simulink library "platooning_custom_blocks"  (R2018b)
settings: Solver=VariableStepAuto  StartTime=0.0  StopTime=10.0  RelTol=1e-3
undefined symbols (not defined in the file): AccPdl_pdlbpt, AccPdl_spdbpt, AccPdl_trqMap, adj_motEffMap, BETModel, BrkPdl_brkTrq, BrkPdl_pdlbpt, Cd_Map, Cd_Map_T2, CT_accPdl_pdlbpt, CT_accPdl_spdbpt, CT_accPdl_trqMap, CT_brkPdl_brkTrq, CT_brkPdl_pdlbpt, CTModel, d_11, d_22, DiscIntNeverNeededParam, init_veh_spd_mps, max_Cd_frac, min_Cd_frac, motSpdVec, motTrqVec, msk_init_pos_m, msk_mot_cont_trq, msk_mot_num, msk_mot_spd_bpt, N_OptResults, sim_t_step, simDrv, SPHETModel, t_step
libraries: simulink x19, $bdroot x16, dspstat3 x2, custom_func x1
(part 4 of 5)

== system platooning_custom_blocks/Series Parallel Hybrid Electric Truck/Series Parallel Hybrid Electric Post-Processing/Distance to Empty Calculator ==
  note: Assuming 10% of the fuel in the tank
      | is not available for consumption.
  blndEC_Wh_m : Inport
  <fuelUsed_L> : Inport  Port=2
  battSOC_frac : Inport  Port=3
  Battery Energy Max : Constant  Value=msk_batt_Ns * msk_batt_Np * msk_batt_Nmod * msk_cell_Vnom * msk_cell_Q_Ah
  Constant : Constant  Value=msk_fuel_init_liters
  Constant1 : Constant  Value=0.2
  Divide : Product  Inputs=*/
  Fuel LHV energy per volume : Constant  Value=msk_fuel_rho_kgpl * msk_fuel_lhv_kwhpkg
  Percent of Fuel in Tank : Gain  Gain=0.9
  Product2 : Product
  Product3 : Product
  Subtract : Sum  Inputs=-+
  Subtract1 : Sum  Inputs=+-
  Subtract2 : Sum  Inputs=++|
  kWh2Wh : Gain  Gain=1000
  m2km : Gain  Gain=0.001
  estDTE_km : Outport
  wires:
  Divide/1 -> m2km/1
  Subtract2/1 -> Divide/1
  kWh2Wh/1 -> Subtract2/2
  Product3/1 -> Subtract2/1
  Subtract1/1 -> Product3/1
  Battery Energy Max/1 -> Product3/2
  Product2/1 -> kWh2Wh/1
  Fuel LHV energy per volume/1 -> Product2/1
  battSOC_frac/1 -> Subtract1/1
  Constant1/1 -> Subtract1/2
  Percent of Fuel in Tank/1 -> Subtract/2
  blndEC_Wh_m/1 -> Divide/2
  <fuelUsed_L>/1 -> Subtract/1
  Subtract/1 -> Product2/2
  Constant/1 -> Percent of Fuel in Tank/1
  m2km/1 -> estDTE_km/1  "estDTE_km"

== system platooning_custom_blocks/Series Parallel Hybrid Electric Truck/Series Parallel Hybrid Electric Post-Processing/Fuel Consumption Calculator ==
  <fuelUsed_L> : Inport
  <DistTrvld_m> : Inport  Port=2
  Constant : Constant  Value=100
  Constant1 : Constant  Value=eps
  Divide1 : Product  Inputs=*/
  Divide2 : Product  Inputs=*/
  Switch : Switch  Criteria=u2 > Threshold
  m2km : Gain  Gain=1/1000
  FC_Lp100km : Outport
  wires:
  Divide2/1 -> FC_Lp100km/1  "FC_Lp100km"
  <DistTrvld_m>/1 -> m2km/1
  Switch/1 -> Divide1/1
  Divide1/1 -> Divide2/2
  m2km/1 -> Switch/1, Switch/2
  <fuelUsed_L>/1 -> Divide1/2
  Constant1/1 -> Switch/3
  Constant/1 -> Divide2/1

== system platooning_custom_blocks/Series Parallel Hybrid Electric Truck/Series Parallel Hybrid Electric Powertrain Power Loss Model/A123 ESS Model ==
  Inp_Current : Inport
  Add : Sum  Inputs=++++
  Bus Creator : BusCreator  Inputs=7
  OCV_Battery : Subsystem
  R0 Resistance : Subsystem
  R1_C1 Circuit : Subsystem
  R2_C2 Circuit : Subsystem
  Info : Outport
  Load_Voltage : Outport  Port=2
  SOC : Outport  Port=3
  Current : Outport  Port=4
  wires:
  [SOC] -> Bus Creator/3
  [U_PA] -> Bus Creator/7
  Inp_Current/1 -> OCV_Battery/1(Current)
  [current] -> Bus Creator/2
  Add/1 -> Load_Voltage/1, [V_L]  "V_L"
  [Em] -> Bus Creator/4
  R0 Resistance/1(V_R0) -> [V_R0], Add/3  "V_R0"
  R2_C2 Circuit/1(U_PA) -> Add/1, [U_PA]  "U_PA"
  OCV_Battery/2(Current_pt) -> Current/1, [current], R2_C2 Circuit/2(Current), R1_C1 Circuit/2(Current), R0 Resistance/2(Current)  "Current"
  OCV_Battery/1(SOC_calc) -> SOC/1, [SOC], R2_C2 Circuit/1(SOC), R1_C1 Circuit/1(SOC), R0 Resistance/1(SOC)  "SOC"
  R1_C1 Circuit/1(U_PC) -> Add/2, [U_PC]  "U_PC"
  [U_PC] -> Bus Creator/6
  OCV_Battery/3(BattVolt_calc) -> [Em], Add/4  "Em"
  [V_R0] -> Bus Creator/5
  Bus Creator/1 -> Info/1  "Info"
  [V_L] -> Bus Creator/1

== system platooning_custom_blocks/Series Parallel Hybrid Electric Truck/Series Parallel Hybrid Electric Powertrain Power Loss Model/Battery EPO Logic ==
  note: Discharge Current is negative
  Batt_SOC_frac : Inport
  LoadCurrent_A : Inport  Port=2
  10-second average : dspstat3/Moving Average  Method=Sliding window  ForgettingFactorPort=off  SpecifyWindowLength=on  WindowLength=1000  ForgettingFactor=0.9  SimulateUsing=Code generation
  10sec Discharge Limit Table A123 : Lookup_n-D  BreakpointsForDimension1=msk_cellTempbpt  BreakpointsForDimension2=msk_soc_bpt  Table=msk_dchglim10s  ExtrapMethod=Clip  UseLastTableValue=on  InternalRulePriority=Speed  RndMeth=Simplest  InputSameDT=on
  Battery EPO Constraint Logic : Stateflow chart  TreatAsAtomicUnit=on
  CellTemp degC : Constant  Value=35
  Gain1 : Gain  Gain=-1
  Batt_EPO : Outport
  wires:
  Batt_SOC_frac/1 -> 10sec Discharge Limit Table A123/2
  LoadCurrent_A/1 -> 10-second average/1
  Battery EPO Constraint Logic/1(epo_flag) -> Batt_EPO/1  "Batt_EPO"
  10-second average/1 -> Battery EPO Constraint Logic/2(LoadCurr)  "LoadCurrent_10sAvg_A"
  CellTemp degC/1 -> 10sec Discharge Limit Table A123/1
  Gain1/1 -> Battery EPO Constraint Logic/1(DchgCurrLim)
  10sec Discharge Limit Table A123/1 -> Gain1/1

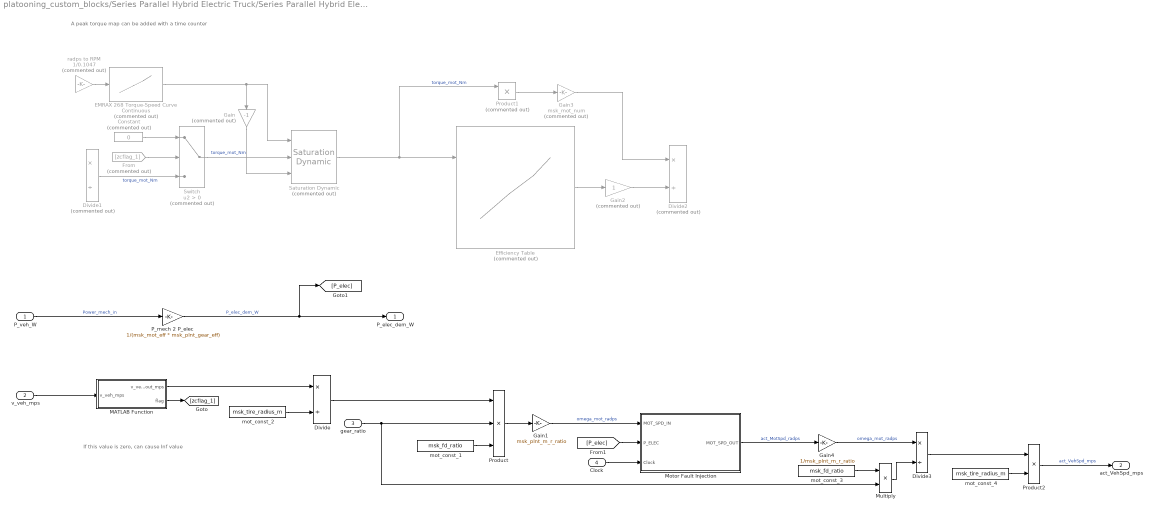
== system platooning_custom_blocks/Series Parallel Hybrid Electric Truck/Series Parallel Hybrid Electric Powertrain Power Loss Model/Electric Drivetrain ==
  note: A peak torque map can be added with a time counter
  note: If this value is zero, can cause Inf value
  P_veh_W : Inport
  v_veh_mps : Inport  Port=2
  gear_ratio : Inport  Port=3
  Clock : Inport  Port=4
  Constant : Constant  Commented=on  Value=0
  Divide : Product  Inputs=*/
  Divide1 : Product  Commented=on  Inputs=*/
  Divide2 : Product  Commented=on  Inputs=*/
  Divide3 : Product  Inputs=*/
  EMRAX 268 Torque-Speed Curve Continuous : Lookup_n-D  Commented=on  NumberOfTableDimensions=1  BreakpointsForDimension1=msk_mot_spd_bpt  Table=msk_mot_cont_trq  InternalRulePriority=Speed  RndMeth=Simplest  InputSameDT=on
  Efficiency Table : Lookup_n-D  Commented=on  BreakpointsForDimension1=motTrqVec  BreakpointsForDimension2=motSpdVec  Table=adj_motEffMap  ExtrapMethod=Clip  UseLastTableValue=on  InternalRulePriority=Speed  RndMeth=Simplest  InputSameDT=on
  From : From  Commented=on  GotoTag=zcflag_1
  Gain : Gain  Commented=on  Gain=-1
  Gain1 : Gain  Gain=msk_plnt_m_r_ratio
  Gain2 : Gain  Commented=on
  Gain3 : Gain  Commented=on  Gain=msk_mot_num
  Gain4 : Gain  Gain=1/msk_plnt_m_r_ratio
  MATLAB Function : MATLAB Function  TreatAsAtomicUnit=on
  Motor Fault Injection : Subsystem  mask{FaultDec=off, P_derate=30000, t_fault=6000, contMotTrqMax=180}
      mask prompts: FaultDec "Select to enable motor deration fault."; P_derate "Enter the motor deration power [Watts]:"; t_fault "Time for fault insertion [seconds]:"; contMotTrqMax "Maximum Continuous Motor Torque [Nm]:"
      mask DialogControl DescGroupVar Prompt: Motor Fault Injection
      mask DialogControl DescTextVar Prompt: Use the parameter controls to induce a deration fault in the motor subsystem.
  Multiply : Product
  P_mech 2 P_elec : Gain  Gain=1/(msk_mot_eff * msk_plnt_gear_eff)
  Product : Product  Inputs=3
  Product1 : Product  Commented=on
  Product2 : Product
  Saturation Dynamic : simulink/Discontinuities/Saturation Dynamic  Commented=on  OutMin=[]  OutMax=[]  OutDataTypeStr=Inherit: Same as second input  OutDataType=fixdt(1, 16)  OutScaling=2^-10  DoSatur=off
  Switch : Switch  Commented=on  Criteria=u2 > Threshold
  mot_const_1 : Constant  Value=msk_fd_ratio
  mot_const_2 : Constant  Value=msk_tire_radius_m
  mot_const_3 : Constant  Value=msk_fd_ratio
  mot_const_4 : Constant  Value=msk_tire_radius_m
  radps to RPM : Gain  Commented=on  Gain=1/0.1047
  P_elec_dem_W : Outport
  act_VehSpd_mps : Outport  Port=2
  wires:
  Saturation Dynamic/1 -> Product1/1, Efficiency Table/1  "torque_mot_Nm"
  From/1 -> Switch/2
  MATLAB Function/1(v_veh_out_mps) -> Divide/1
  radps to RPM/1 -> EMRAX 268 Torque-Speed Curve Continuous/1
  Constant/1 -> Switch/1
  Gain/1 -> Saturation Dynamic/3
  gear_ratio/1 -> Multiply/2, Product/2
  EMRAX 268 Torque-Speed Curve Continuous/1 -> Gain/1, Saturation Dynamic/1
  P_veh_W/1 -> P_mech 2 P_elec/1  "Power_mech_in"
  v_veh_mps/1 -> MATLAB Function/1(v_veh_mps)
  Efficiency Table/1 -> Gain2/1
  Switch/1 -> Saturation Dynamic/2  "torque_mot_Nm"
  mot_const_2/1 -> Divide/2
  MATLAB Function/2(flag) -> [zcflag_1]
  Product1/1 -> Gain3/1
  P_mech 2 P_elec/1 -> [P_elec], P_elec_dem_W/1  "P_elec_dem_W"
  Gain2/1 -> Divide2/2
  Gain3/1 -> Divide2/1
  Divide1/1 -> Switch/3  "torque_mot_Nm"
  Motor Fault Injection/1(MOT_SPD_OUT) -> Gain4/1  "act_MotSpd_radps"
  Gain1/1 -> Motor Fault Injection/1(MOT_SPD_IN)  "omega_mot_radps"
  [P_elec] -> Motor Fault Injection/2(P_ELEC)
  Clock/1 -> Motor Fault Injection/3(Clock)
  mot_const_3/1 -> Multiply/1
  Divide3/1 -> Product2/1
  mot_const_4/1 -> Product2/2
  Product2/1 -> act_VehSpd_mps/1  "act_VehSpd_mps"
  Divide/1 -> Product/1
  mot_const_1/1 -> Product/3
  Product/1 -> Gain1/1
  Gain4/1 -> Divide3/1  "omega_mot_radps"
  Multiply/1 -> Divide3/2

== system platooning_custom_blocks/Series Parallel Hybrid Electric Truck/Series Parallel Hybrid Electric Powertrain Power Loss Model/Engine Torque Saturation ==
  eng_brk_trq : Inport
  eng_spd_rpm : Inport  Port=2
  Engine Peak Motoring Torque LUT : Lookup_n-D  NumberOfTableDimensions=1  BreakpointsForDimension1=msk_eng_trq_spd_bpt  Table=msk_eng_pk_mtr_trq  ExtrapMethod=Clip  UseLastTableValue=on  InternalRulePriority=Speed  RndMeth=Simplest  InputSameDT=on
  "Engine Peak Propulsion Torque LUT " : Lookup_n-D  NumberOfTableDimensions=1  BreakpointsForDimension1=msk_eng_trq_spd_bpt  Table=msk_eng_pk_trq_vec  ExtrapMethod=Clip  UseLastTableValue=on  InternalRulePriority=Speed  RndMeth=Simplest  InputSameDT=on
  Saturation Dynamic : simulink/Discontinuities/Saturation Dynamic  OutMin=[]  OutMax=[]  OutDataTypeStr=Inherit: Same as second input  OutDataType=fixdt(1, 16)  OutScaling=2^-10  DoSatur=off
  eng_brk_trq_out : Outport
  wires:
  eng_brk_trq/1 -> Saturation Dynamic/2
  Saturation Dynamic/1 -> eng_brk_trq_out/1
  eng_spd_rpm/1 -> "Engine Peak Propulsion Torque LUT "/1, Engine Peak Motoring Torque LUT/1
  Engine Peak Motoring Torque LUT/1 -> Saturation Dynamic/3
  "Engine Peak Propulsion Torque LUT "/1 -> Saturation Dynamic/1

== system platooning_custom_blocks/Series Parallel Hybrid Electric Truck/Series Parallel Hybrid Electric Powertrain Power Loss Model/Fuel Level Calculator ==
  mfuel_gps : Inport
  Constant : Constant  Value=msk_fuel_init_liters
  Discrete-Time Integrator : DiscreteIntegrator  SampleTime=msk_t_step  ICPrevOutput=DiscIntNeverNeededParam  ICPrevScaledInput=DiscIntNeverNeededParam
  Divide1 : Product  Inputs=*/
  Fuel Density : Gain  Gain=(0.001/msk_rho_fuel_kgpL)
  Gain1 : Gain  Gain=100
  Subtract : Sum  Inputs=+-
  fuelLvl_pct : Outport
  fuelUsed_L : Outport  Port=2
  wires:
  Divide1/1 -> Gain1/1
  Subtract/1 -> Divide1/1  "fuelLeft_liters"
  Fuel Density/1 -> fuelUsed_L/1, Subtract/2  "fuelUsed_liters"
  Constant/1 -> Divide1/2, Subtract/1
  Discrete-Time Integrator/1 -> Fuel Density/1  "mfuel_g"
  mfuel_gps/1 -> Discrete-Time Integrator/1
  Gain1/1 -> fuelLvl_pct/1  "fuelLvl_pct"

== system platooning_custom_blocks/Series Parallel Hybrid Electric Truck/Series Parallel Hybrid Electric Truck Energy Management System/Battery Power Limit Calculator ==
  <Batt_SOC_frac> : Inport
  <Batt_Voltage_V> : Inport  Port=2
  Battery Continuous Charge Limit : Lookup_n-D  BreakpointsForDimension1=SPHETModel.cellTempbpt_C  BreakpointsForDimension2=SPHETModel.socbpt  Table=SPHETModel.ChgCurrLim_cont_A  ExtrapMethod=Clip  UseLastTableValue=on  InternalRulePriority=Speed  RndMeth=Simplest  InputSameDT=on
  Constant3 : Constant  Value=25
  Gain1 : Gain
  Multiply : Product
  P_BattChgContLim : Outport
  wires:
  Multiply/1 -> P_BattChgContLim/1  "P_BattChgContLim"
  <Batt_SOC_frac>/1 -> Battery Continuous Charge Limit/2
  Battery Continuous Charge Limit/1 -> Gain1/1
  Gain1/1 -> Multiply/1
  Constant3/1 -> Battery Continuous Charge Limit/1
  <Batt_Voltage_V>/1 -> Multiply/2

== system platooning_custom_blocks/Series Parallel Hybrid Electric Truck/Series Parallel Hybrid Electric Truck Energy Management System/Generator Power Limit Calculator ==
  gen_spd_rpm : Inport
  Constant : Constant  Value=5000
  Divide : Product  Inputs=*/
  Gain : Gain
  Generator Continuous Power kW : Lookup_n-D  NumberOfTableDimensions=1  BreakpointsForDimension1=SPHETModel.cont_gen_mtr_trq_spdbpt  Table=SPHETModel.cont_gen_mtr_pwr_map  ExtrapMethod=Clip  UseLastTableValue=on  InternalRulePriority=Speed  RndMeth=Simplest  InputSameDT=on
  Generator Continuous Torque : Lookup_n-D  NumberOfTableDimensions=1  BreakpointsForDimension1=SPHETModel.cont_gen_mtr_trq_spdbpt  Table=SPHETModel.cont_gen_mtr_trq_map  ExtrapMethod=Clip  UseLastTableValue=on  InternalRulePriority=Speed  RndMeth=Simplest  InputSameDT=on
  Generator Efficiency : Lookup_n-D  BreakpointsForDimension1=SPHETModel.gen_mtr_trqbpt  BreakpointsForDimension2=SPHETModel.gen_mtr_spdbpt  Table=SPHETModel.gen_mtr_eff_map  ExtrapMethod=Clip  UseLastTableValue=on  InternalRulePriority=Speed  RndMeth=Simplest  InputSameDT=on
  kW2W : Gain  Gain=1000
  P_GenMtrContLim : Outport
  wires:
  Constant/1 -> Generator Continuous Power kW/1
  Gain/1 -> P_GenMtrContLim/1
  Divide/1 -> Gain/1  "P_GenMtrContLim"
  Generator Continuous Torque/1 -> Generator Efficiency/1
  Generator Efficiency/1 -> Divide/2
  Generator Continuous Power kW/1 -> kW2W/1
  kW2W/1 -> Divide/1
  gen_spd_rpm/1 -> Generator Efficiency/2, Generator Continuous Torque/1

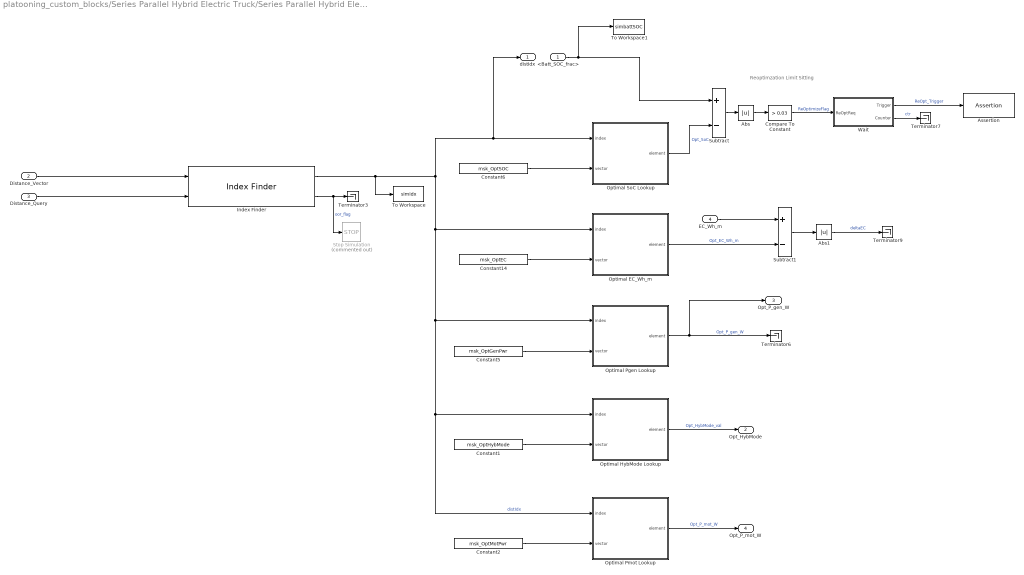
== system platooning_custom_blocks/Series Parallel Hybrid Electric Truck/Series Parallel Hybrid Electric Truck Energy Management System/Proposed ReOpt DP Algorithm ==
  note: Reoptimzation Limit Sitting
  <Batt_SOC_frac> : Inport
  Distance_Vector : Inport  Port=2
  Distance_Query : Inport  Port=3
  EC_Wh_m : Inport  Port=4
  Abs : Abs
  Abs1 : Abs
  Assertion : Assertion  AssertionFailFcn=set_param(bdroot,'SimulationCommand','pause');  StopWhenAssertionFail=off
  Compare To Constant : simulink/Logic and Bit Operations/Compare To Constant  relop=>  const=0.03  OutDataTypeStr=boolean
  Constant1 : Constant  Value=msk_OptHybMode
  Constant14 : Constant  Value=msk_OptEC
  Constant2 : Constant  Value=msk_OptMotPwr
  Constant5 : Constant  Value=msk_OptGenPwr
  Constant6 : Constant  Value=msk_OptSOC
  Index Finder : custom_func/Index Finder  SystemSampleTime=-1
  Optimal EC_Wh_m : MATLAB Function  TreatAsAtomicUnit=on
  Optimal HybMode Lookup : MATLAB Function  TreatAsAtomicUnit=on
  Optimal Pgen Lookup : MATLAB Function  TreatAsAtomicUnit=on
  Optimal Pmot Lookup : MATLAB Function  TreatAsAtomicUnit=on
  Optimal SoC Lookup : MATLAB Function  TreatAsAtomicUnit=on
  Stop Simulation : Stop  Commented=on
  Subtract : Sum  Inputs=+-
  Subtract1 : Sum  Inputs=+-
  Terminator{3,6..7,9} (4 alike) : Terminator
  To Workspace : ToWorkspace  VariableName=simidx  SaveFormat=Timeseries  SampleTime=1
      settings: Save2DSignal=2-D array (concatenate along first dimension)
  To Workspace1 : ToWorkspace  VariableName=simbattSOC  SaveFormat=Timeseries  SampleTime=1
      settings: Save2DSignal=2-D array (concatenate along first dimension)
  Wait : Stateflow chart  TreatAsAtomicUnit=on
  distIdx : Outport
  Opt_HybMode : Outport  Port=2
  Opt_P_gen_W : Outport  Port=3
  Opt_P_mot_W : Outport  Port=4
  wires:
  Optimal HybMode Lookup/1(element) -> Opt_HybMode/1  "Opt_HybMode_val"
  Optimal Pmot Lookup/1(element) -> Opt_P_mot_W/1  "Opt_P_mot_W"
  Constant2/1 -> Optimal Pmot Lookup/2(vector)
  Constant1/1 -> Optimal HybMode Lookup/2(vector)
  Constant14/1 -> Optimal EC_Wh_m/2(vector)
  Wait/1(Trigger) -> Assertion/1  "ReOpt_Trigger"
  Constant5/1 -> Optimal Pgen Lookup/2(vector)
  Index Finder/2 -> Stop Simulation/1, Terminator3/1  "oor_flag"
  Optimal Pgen Lookup/1(element) -> Terminator6/1, Opt_P_gen_W/1  "Opt_P_gen_W"
  Wait/2(Counter) -> Terminator7/1  "ctr"
  Subtract1/1 -> Abs1/1
  Optimal EC_Wh_m/1(element) -> Subtract1/2  "Opt_EC_Wh_m"
  Optimal SoC Lookup/1(element) -> Subtract/2  "Opt_SoC"
  EC_Wh_m/1 -> Subtract1/1
  Index Finder/1 -> Optimal Pgen Lookup/1(index), Optimal Pmot Lookup/1(index), Optimal HybMode Lookup/1(index), Optimal EC_Wh_m/1(index), Optimal SoC Lookup/1(index), distIdx/1, To Workspace/1  "distIdx"
  Abs/1 -> Compare To Constant/1
  Compare To Constant/1 -> Wait/1(ReOptReq)  "ReOptimizeFlag"
  Constant6/1 -> Optimal SoC Lookup/2(vector)
  Subtract/1 -> Abs/1
  Distance_Vector/1 -> Index Finder/1
  Abs1/1 -> Terminator9/1  "deltaEC"
  <Batt_SOC_frac>/1 -> Subtract/1, To Workspace1/1
  Distance_Query/1 -> Index Finder/2

== system platooning_custom_blocks/Series Parallel Hybrid Electric Truck/Series Parallel Hybrid Electric Truck Energy Management System/SPHET Optimal Gear Shift Algorithm ==
  P_dem_W : Inport
  veh_spd_mps : Inport  Port=2
  Bus Creator : BusCreator  Inputs=10
  Constant : Constant  Value=eps
  Divide : Product  Inputs=*/
  Fuel LUT @ Gear 1 : Lookup_n-D  BreakpointsForDimension1=CTModel.eng_map_trq_bpt(10:end) * (CTModel.gear_ratios(1) * CTModel.fd_ratio)  BreakpointsForDimension2=(CTModel.eng_map_spd_bpt * 0.1047 * CTModel.ld_tire_rad_m)/(CTModel.gear_ratios(1) * CTModel.fd_ratio)  Table=CTModel.eng_fuel_map(10:end,:)  ExtrapMethod=Clip  UseLastTableValue=on  InternalRulePriority=Speed  RndMeth=Simplest  InputSameDT=on
  Fuel LUT @ Gear 10 : Lookup_n-D  BreakpointsForDimension1=CTModel.eng_map_trq_bpt(10:end) * (CTModel.gear_ratios(10) * CTModel.fd_ratio)  BreakpointsForDimension2=(CTModel.eng_map_spd_bpt * 0.1047 * CTModel.ld_tire_rad_m)/(CTModel.gear_ratios(10) * CTModel.fd_ratio)  Table=CTModel.eng_fuel_map(10:end,:)  ExtrapMethod=Clip  UseLastTableValue=on  InternalRulePriority=Speed  RndMeth=Simplest  InputSameDT=on
  Fuel LUT @ Gear 2 : Lookup_n-D  BreakpointsForDimension1=CTModel.eng_map_trq_bpt(10:end) * (CTModel.gear_ratios(2) * CTModel.fd_ratio)  BreakpointsForDimension2=(CTModel.eng_map_spd_bpt * 0.1047 * CTModel.ld_tire_rad_m)/(CTModel.gear_ratios(2) * CTModel.fd_ratio)  Table=CTModel.eng_fuel_map(10:end,:)  ExtrapMethod=Clip  UseLastTableValue=on  InternalRulePriority=Speed  RndMeth=Simplest  InputSameDT=on
  Fuel LUT @ Gear 3 : Lookup_n-D  BreakpointsForDimension1=CTModel.eng_map_trq_bpt(10:end) * (CTModel.gear_ratios(3) * CTModel.fd_ratio)  BreakpointsForDimension2=(CTModel.eng_map_spd_bpt * 0.1047 * CTModel.ld_tire_rad_m)/(CTModel.gear_ratios(3) * CTModel.fd_ratio)  Table=CTModel.eng_fuel_map(10:end,:)  ExtrapMethod=Clip  UseLastTableValue=on  InternalRulePriority=Speed  RndMeth=Simplest  InputSameDT=on
  Fuel LUT @ Gear 4 : Lookup_n-D  BreakpointsForDimension1=CTModel.eng_map_trq_bpt(10:end) * (CTModel.gear_ratios(4) * CTModel.fd_ratio)  BreakpointsForDimension2=(CTModel.eng_map_spd_bpt * 0.1047 * CTModel.ld_tire_rad_m)/(CTModel.gear_ratios(4) * CTModel.fd_ratio)  Table=CTModel.eng_fuel_map(10:end,:)  ExtrapMethod=Clip  UseLastTableValue=on  InternalRulePriority=Speed  RndMeth=Simplest  InputSameDT=on
  Fuel LUT @ Gear 5 : Lookup_n-D  BreakpointsForDimension1=CTModel.eng_map_trq_bpt(10:end) * (CTModel.gear_ratios(5) * CTModel.fd_ratio)  BreakpointsForDimension2=(CTModel.eng_map_spd_bpt * 0.1047 * CTModel.ld_tire_rad_m)/(CTModel.gear_ratios(5) * CTModel.fd_ratio)  Table=CTModel.eng_fuel_map(10:end,:)  ExtrapMethod=Clip  UseLastTableValue=on  InternalRulePriority=Speed  RndMeth=Simplest  InputSameDT=on
  Fuel LUT @ Gear 6 : Lookup_n-D  BreakpointsForDimension1=CTModel.eng_map_trq_bpt(10:end) * (CTModel.gear_ratios(6) * CTModel.fd_ratio)  BreakpointsForDimension2=(CTModel.eng_map_spd_bpt * 0.1047 * CTModel.ld_tire_rad_m)/(CTModel.gear_ratios(6) * CTModel.fd_ratio)  Table=CTModel.eng_fuel_map(10:end,:)  ExtrapMethod=Clip  UseLastTableValue=on  InternalRulePriority=Speed  RndMeth=Simplest  InputSameDT=on
  Fuel LUT @ Gear 7 : Lookup_n-D  BreakpointsForDimension1=CTModel.eng_map_trq_bpt(10:end) * (CTModel.gear_ratios(7) * CTModel.fd_ratio)  BreakpointsForDimension2=(CTModel.eng_map_spd_bpt * 0.1047 * CTModel.ld_tire_rad_m)/(CTModel.gear_ratios(7) * CTModel.fd_ratio)  Table=CTModel.eng_fuel_map(10:end,:)  ExtrapMethod=Clip  UseLastTableValue=on  InternalRulePriority=Speed  RndMeth=Simplest  InputSameDT=on
  Fuel LUT @ Gear 8 : Lookup_n-D  BreakpointsForDimension1=CTModel.eng_map_trq_bpt(10:end) * (CTModel.gear_ratios(8) * CTModel.fd_ratio)  BreakpointsForDimension2=(CTModel.eng_map_spd_bpt * 0.1047 * CTModel.ld_tire_rad_m)/(CTModel.gear_ratios(8) * CTModel.fd_ratio)  Table=CTModel.eng_fuel_map(10:end,:)  ExtrapMethod=Clip  UseLastTableValue=on  InternalRulePriority=Speed  RndMeth=Simplest  InputSameDT=on
  Fuel LUT @ Gear 9 : Lookup_n-D  BreakpointsForDimension1=CTModel.eng_map_trq_bpt(10:end) * (CTModel.gear_ratios(9) * CTModel.fd_ratio)  BreakpointsForDimension2=(CTModel.eng_map_spd_bpt * 0.1047 * CTModel.ld_tire_rad_m)/(CTModel.gear_ratios(9) * CTModel.fd_ratio)  Table=CTModel.eng_fuel_map(10:end,:)  ExtrapMethod=Clip  UseLastTableValue=on  InternalRulePriority=Speed  RndMeth=Simplest  InputSameDT=on
  Loaded Tire Radius m : Gain  Gain=msk_tire_radius_m
  Minimum Function : MATLAB Function  TreatAsAtomicUnit=on
  Switch : Switch  Criteria=u2 > Threshold
  Transmission Efficiency : Gain  Gain=1/msk_trns_eff_avg
  init_gear : Constant  Value=msk_init_gear
  opt_gear : Outport
  wires:
  Fuel LUT @ Gear 4/1 -> Bus Creator/4  "m_fuel_Gear_4"
  Loaded Tire Radius m/1 -> Transmission Efficiency/1
  init_gear/1 -> Minimum Function/2(prev_gear)
  veh_spd_mps/1 -> Switch/2, Switch/1, Fuel LUT @ Gear 1/2, Fuel LUT @ Gear 10/2, Fuel LUT @ Gear 9/2, Fuel LUT @ Gear 8/2, Fuel LUT @ Gear 7/2, Fuel LUT @ Gear 6/2, Fuel LUT @ Gear 5/2, Fuel LUT @ Gear 4/2, Fuel LUT @ Gear 3/2, Fuel LUT @ Gear 2/2
  Constant/1 -> Switch/3
  Fuel LUT @ Gear 1/1 -> Bus Creator/1  "m_fuel_Gear_1"
  Fuel LUT @ Gear 7/1 -> Bus Creator/7  "m_fuel_Gear_7"
  Minimum Function/1(opt_gear) -> opt_gear/1
  Fuel LUT @ Gear 10/1 -> Bus Creator/10  "m_fuel_Gear_10"
  Switch/1 -> Divide/2
  Fuel LUT @ Gear 3/1 -> Bus Creator/3  "m_fuel_Gear_3"
  Divide/1 -> Fuel LUT @ Gear 10/1, Fuel LUT @ Gear 9/1, Fuel LUT @ Gear 8/1, Fuel LUT @ Gear 7/1, Fuel LUT @ Gear 6/1, Fuel LUT @ Gear 5/1, Fuel LUT @ Gear 4/1, Fuel LUT @ Gear 3/1, Fuel LUT @ Gear 2/1, Fuel LUT @ Gear 1/1
  Fuel LUT @ Gear 9/1 -> Bus Creator/9  "m_fuel_Gear_9"
  Fuel LUT @ Gear 8/1 -> Bus Creator/8  "m_fuel_Gear_8"
  Fuel LUT @ Gear 2/1 -> Bus Creator/2  "m_fuel_Gear_2"
  Bus Creator/1 -> Minimum Function/1(m_fuel_vec)
  Fuel LUT @ Gear 6/1 -> Bus Creator/6  "m_fuel_Gear_6"
  Fuel LUT @ Gear 5/1 -> Bus Creator/5  "m_fuel_Gear_5"
  P_dem_W/1 -> Loaded Tire Radius m/1
  Transmission Efficiency/1 -> Divide/1

== system platooning_custom_blocks/Battery Electric Truck/Battery Electric Powertrain Power Loss Model/A123 ESS Model/OCV_Battery ==
  note: Intial SOC value goes in this memory block
  Current : Inport
  Add : Sum
  Constant : Constant  Value=msk_batt_Ns
  Constant1 : Constant  Value=msk_cell_Q_Ah * msk_batt_Np
  Constant2 : Constant  Value=msk_batt_Nmod
  Divide : Product  Inputs=*/
  Gain : Gain  Gain=msk_t_step/3600
  Memory : Memory  InitialCondition=msk_batt_soc_init  InheritSampleTime=on  LinearizeAsDelay=on
  OCV Function : MATLAB Function  TreatAsAtomicUnit=on
  Product : Product  Inputs=3
  Unit Delay : UnitDelay  SampleTime=-1
  SOC_calc : Outport
  Current_pt : Outport  Port=2
  BattVolt_calc : Outport  Port=3
  wires:
  Unit Delay/1 -> Product/1  "OCV_calc"
  Current/1 -> OCV Function/2(current), Current_pt/1, Gain/1
  Gain/1 -> Divide/1
  Memory/1 -> Add/1
  Constant2/1 -> Product/3
  OCV Function/1(ocv) -> Unit Delay/1
  Constant1/1 -> Divide/2
  Add/1 -> SOC_calc/1, Memory/1, OCV Function/1(soc)  "SOC_calc"
  Constant/1 -> Product/2
  Divide/1 -> Add/2
  Product/1 -> BattVolt_calc/1  "BattVolt_calc"

== system platooning_custom_blocks/Battery Electric Truck/Battery Electric Powertrain Power Loss Model/A123 ESS Model/R0 Resistance ==
  SOC : Inport
  Current : Inport  Port=2
  Compare To Zero : simulink/Logic and Bit Operations/Compare To Zero  relop=>  OutDataTypeStr=boolean
  Product : Product
  R0 LUT Chg : Lookup_n-D  NumberOfTableDimensions=1  BreakpointsForDimension1=msk_batt_soc_bpt  Table=msk_batt_R0 * 0.05  InternalRulePriority=Speed  RndMeth=Simplest  InputSameDT=on
  R0 LUT Dchg : Lookup_n-D  NumberOfTableDimensions=1  BreakpointsForDimension1=msk_batt_soc_bpt  Table=msk_batt_R0 * 0.25  InternalRulePriority=Speed  RndMeth=Simplest  InputSameDT=on
  Switch : Switch  Criteria=u2 > Threshold
  V_R0 : Outport
  wires:
  R0 LUT Chg/1 -> Switch/1  "R0"
  SOC/1 -> R0 LUT Chg/1, R0 LUT Dchg/1
  Current/1 -> Compare To Zero/1, Product/2
  Product/1 -> V_R0/1
  Switch/1 -> Product/1
  Compare To Zero/1 -> Switch/2
  R0 LUT Dchg/1 -> Switch/3  "R0"

== system platooning_custom_blocks/Battery Electric Truck/Battery Electric Powertrain Power Loss Model/A123 ESS Model/R1_C1 Circuit ==
  SOC : Inport
  Current : Inport  Port=2
  Add1 : Sum
  C1 LUT : Lookup_n-D  NumberOfTableDimensions=1  BreakpointsForDimension1=msk_batt_soc_bpt  Table=msk_batt_C1  InternalRulePriority=Speed  RndMeth=Simplest  InputSameDT=on
  Discrete-Time Integrator : DiscreteIntegrator  SampleTime=-1  ICPrevOutput=DiscIntNeverNeededParam  ICPrevScaledInput=DiscIntNeverNeededParam
  Divide : Product  Inputs=*/
  Divide1 : Product  Inputs=*/
  Product : Product
  R1 LUT : Lookup_n-D  NumberOfTableDimensions=1  BreakpointsForDimension1=msk_batt_soc_bpt  Table=msk_batt_R1  InternalRulePriority=Speed  RndMeth=Simplest  InputSameDT=on
  U_PC : Outport
  wires:
  Product/1 -> Divide1/2
  SOC/1 -> R1 LUT/1, C1 LUT/1
  Divide1/1 -> Add1/1
  C1 LUT/1 -> Product/2, Divide/2
  Divide/1 -> Add1/2
  R1 LUT/1 -> Product/1
  Discrete-Time Integrator/1 -> U_PC/1, Divide1/1  "U_PC"
  Add1/1 -> Discrete-Time Integrator/1  "U_PC_derivative"
  Current/1 -> Divide/1

== system platooning_custom_blocks/Battery Electric Truck/Battery Electric Powertrain Power Loss Model/A123 ESS Model/R2_C2 Circuit ==
  SOC : Inport
  Current : Inport  Port=2
  Add1 : Sum
  C2 LUT : Lookup_n-D  NumberOfTableDimensions=1  BreakpointsForDimension1=msk_batt_soc_bpt  Table=msk_batt_C2  InternalRulePriority=Speed  RndMeth=Simplest  InputSameDT=on
  Discrete-Time Integrator : DiscreteIntegrator  SampleTime=-1  ICPrevOutput=DiscIntNeverNeededParam  ICPrevScaledInput=DiscIntNeverNeededParam
  Divide : Product  Inputs=*/
  Divide1 : Product  Inputs=*/
  Product : Product
  R2 LUT : Lookup_n-D  NumberOfTableDimensions=1  BreakpointsForDimension1=msk_batt_soc_bpt  Table=msk_batt_R2  InternalRulePriority=Speed  RndMeth=Simplest  InputSameDT=on
  U_PA : Outport
  wires:
  Product/1 -> Divide1/2
  SOC/1 -> R2 LUT/1, C2 LUT/1
  Divide1/1 -> Add1/1
  C2 LUT/1 -> Product/2, Divide/2
  Divide/1 -> Add1/2
  R2 LUT/1 -> Product/1
  Discrete-Time Integrator/1 -> U_PA/1, Divide1/1  "U_PA"
  Add1/1 -> Discrete-Time Integrator/1  "U_PA_derivative"
  Current/1 -> Divide/1

== system platooning_custom_blocks/Battery Electric Truck/Battery Electric Powertrain Power Loss Model/Electric Drivetrain/Motor Fault Injection ==
  MOT_SPD_IN : Inport
  P_ELEC : Inport  Port=2
  Clock : Inport  Port=3
  Add : Sum  Inputs=|-+
  Add1 : Sum
  Constant : Constant  Value=t_fault
  Constant1 : Constant  Value=0
  Constant2 : Constant  Value=contMotTrqMax
  Delay : Delay  DelayLength=1
  Discrete PID Controller : simulink/Continuous/PID Controller  Controller=PI  Form=Parallel  TimeDomain=Discrete-time  SampleTime=-1  IntegratorMethod=Forward Euler  FilterMethod=Forward Euler  ControllerParametersSource=internal  P=0.002  I=0.003  D=0  UseFilter=on  N=100  TunerSelectOption=Transfer Function Based (PID Tuner App)  InitialConditionSource=internal  InitialConditionForIntegrator=0  InitialConditionForFilter=0  DifferentiatorICPrevScaledInput=0  ExternalReset=none  TrackingMode=off  Kt=1  LimitOutput=on  UpperSaturationLimit=0  LowerSaturationLimit=-inf  LinearizeAsGain=off  AntiWindupMode=clamping  Kb=1  POutMin=[]  POutMax=[]  IOutMin=[]  IOutMax=[]  DOutMin=[]  DOutMax=[]  NOutMin=[]  NOutMax=[]  SumOutMin=[]  SumOutMax=[]  SaturationOutMin=[]  SaturationOutMax=[]  PParamMin=[]  PParamMax=[]  IParamMin=[]  IParamMax=[]  DParamMin=[]  DParamMax=[]  NParamMin=[]  NParamMax=[]  KbParamMin=[]  KbParamMax=[]  KtParamMin=[]  KtParamMax=[]  KbOutMin=[]  KbOutMax=[]  KtOutMin=[]  KtOutMax=[]  IntegratorOutMin=[]  IntegratorOutMax=[]  FilterOutMin=[]  FilterOutMax=[]  SumI1OutMin=[]  SumI1OutMax=[]  SumI2OutMin=[]  SumI2OutMax=[]  SumI3OutMin=[]  SumI3OutMax=[]  SumI4OutMin=[]  SumI4OutMax=[]  SumDOutMin=[]  SumDOutMax=[]  DifferentiatorOutMin=[]  DifferentiatorOutMax=[]  FilterDiffOutCoefMin=[]  FilterDiffOutCoefMax=[]  ReciprocalOutMin=[]  ReciprocalOutMax=[]  SumDenOutMin=[]  SumDenOutMax=[]  SumNumOutMin=[]  SumNumOutMax=[]  DivideOutMin=[]  DivideOutMax=[]  IntegratorContinuousStateAttributes=''  IntegratorStateMustResolveToSignalObject=off  IntegratorRTWStateStorageClass=Auto  FilterContinuousStateAttributes=''  FilterStateMustResolveToSignalObject=off  FilterRTWStateStorageClass=Auto  ParallelPVariant=InternalParameters  IdealPVariant=Disabled  IVariant=InternalParameters  DVariant=Disabled  IntegratorVariant=Discrete  SatVariant=Enabled  AWVariant=DiscClampingParallel  PCopyVariant=Disabled  TRVariant=Disabled  FdbkBlocksVariant=Forward  IdealPFdbkVariant=Disabled  SatFdbkVariant=Disabled  DerivativeFilterVariant=Disabled  NVariant=Disabled  NCopyVariant=Disabled_SignalSpec  FilterICVariant=Disabled  IntegratorICVariant=InternalICs  ExternalResetVariant=Disabled  TRSumVariant=Passthrough  SumFdbkVariant=Disabled  SumVariant=Sum_PI
  Divide : Product  Inputs=*/
  Equal : RelationalOperator  OutDataTypeStr=boolean  RndMeth=Simplest
  Fault Assertion : Assertion  Commented=on  AssertionFailFcn=|  StopWhenAssertionFail=off
      | set_param(bdroot,'SimulationCommand','pause');
      | disp('## Paused due to Motor fault insertion')
  Gain : Gain  Gain=2
  Logic : Stateflow chart  TreatAsAtomicUnit=on
  Multiport Switch : MultiPortSwitch  DataPortOrder=Zero-based contiguous  Inputs=2  zeroidx=on
  P_ref : Constant  Value=P_derate/2
  P_ref1 : Constant  Value=inf
  Saturation Dynamic : simulink/Discontinuities/Saturation Dynamic  OutMin=[]  OutMax=[]  OutDataTypeStr=Inherit: Same as second input  OutDataType=fixdt(1, 16)  OutScaling=2^-10  DoSatur=off
  Switch : Switch  Criteria=u2 > Threshold
  Switch1 : Switch  Criteria=u2 > Threshold
  choice : Constant  Value=FaultDec
  MOT_SPD_OUT : Outport
  wires:
  Multiport Switch/1 -> MOT_SPD_OUT/1  "omega_mot_radps"
  choice/1 -> Logic/2(choice), Multiport Switch/1
  Add/1 -> Discrete PID Controller/1
  P_ELEC/1 -> Delay/1
  Delay/1 -> Add/1
  Discrete PID Controller/1 -> Add1/2  "PI_Out"
  MOT_SPD_IN/1 -> Multiport Switch/2, Add1/1
  P_ref/1 -> Gain/1, Switch/1
  Saturation Dynamic/1 -> Multiport Switch/3  "omega_mot_radps"
  Add1/1 -> Saturation Dynamic/2  "omega_mot_radps"
  Clock/1 -> Equal/1
  Constant/1 -> Equal/2
  Equal/1 -> Logic/1(input), Switch1/2, Switch/2
  Switch/1 -> Add/2
  P_ref1/1 -> Switch1/3, Switch/3
  Constant1/1 -> Saturation Dynamic/3
  Gain/1 -> Divide/1
  Constant2/1 -> Divide/2
  Divide/1 -> Switch1/1  "max_omega_derate"
  Switch1/1 -> Saturation Dynamic/1
  Logic/1(trigger) -> Fault Assertion/1  "faultTrigger"

== system platooning_custom_blocks/Series Parallel Hybrid Electric Truck/Series Parallel Hybrid Electric Powertrain Power Loss Model/A123 ESS Model/OCV_Battery ==
  note: Intial SOC value goes in this memory block
  Current : Inport
  Add : Sum
  Constant : Constant  Value=msk_batt_Ns
  Constant1 : Constant  Value=msk_cell_Q_Ah * msk_batt_Np
  Constant2 : Constant  Value=msk_batt_Nmod
  Divide : Product  Inputs=*/
  Gain : Gain  Gain=msk_t_step/3600
  Memory : Memory  InitialCondition=msk_batt_soc_init  InheritSampleTime=on  LinearizeAsDelay=on
  OCV Function : MATLAB Function  TreatAsAtomicUnit=on
  Product : Product  Inputs=3
  SOC_calc : Outport
  Current_pt : Outport  Port=2
  BattVolt_calc : Outport  Port=3
  wires:
  Current/1 -> OCV Function/2(current), Current_pt/1, Gain/1
  Gain/1 -> Divide/1
  Memory/1 -> Add/1
  Constant2/1 -> Product/3
  OCV Function/1(ocv) -> Product/1  "OCV_calc"
  Constant1/1 -> Divide/2
  Add/1 -> SOC_calc/1, Memory/1, OCV Function/1(soc)  "SOC_calc"
  Constant/1 -> Product/2
  Divide/1 -> Add/2
  Product/1 -> BattVolt_calc/1  "BattVolt_calc"

== system platooning_custom_blocks/Series Parallel Hybrid Electric Truck/Series Parallel Hybrid Electric Powertrain Power Loss Model/A123 ESS Model/R0 Resistance ==
  SOC : Inport
  Current : Inport  Port=2
  Compare To Zero : simulink/Logic and Bit Operations/Compare To Zero  relop=>  OutDataTypeStr=boolean
  Product : Product
  R0 LUT Chg : Lookup_n-D  NumberOfTableDimensions=1  BreakpointsForDimension1=msk_batt_soc_bpt  Table=msk_batt_R0 * 0.05  ExtrapMethod=Clip  UseLastTableValue=on  InternalRulePriority=Speed  RndMeth=Simplest  InputSameDT=on
  R0 LUT Dchg : Lookup_n-D  NumberOfTableDimensions=1  BreakpointsForDimension1=msk_batt_soc_bpt  Table=msk_batt_R0 * 0.25  ExtrapMethod=Clip  UseLastTableValue=on  InternalRulePriority=Speed  RndMeth=Simplest  InputSameDT=on
  Switch : Switch  Criteria=u2 > Threshold
  V_R0 : Outport
  wires:
  R0 LUT Chg/1 -> Switch/1  "R0"
  SOC/1 -> R0 LUT Chg/1, R0 LUT Dchg/1
  Current/1 -> Compare To Zero/1, Product/2
  Product/1 -> V_R0/1
  Switch/1 -> Product/1
  Compare To Zero/1 -> Switch/2
  R0 LUT Dchg/1 -> Switch/3  "R0"

== system platooning_custom_blocks/Series Parallel Hybrid Electric Truck/Series Parallel Hybrid Electric Powertrain Power Loss Model/A123 ESS Model/R1_C1 Circuit ==
  SOC : Inport
  Current : Inport  Port=2
  Add1 : Sum
  C1 LUT : Lookup_n-D  NumberOfTableDimensions=1  BreakpointsForDimension1=msk_batt_soc_bpt  Table=msk_batt_C1  ExtrapMethod=Clip  UseLastTableValue=on  InternalRulePriority=Speed  RndMeth=Simplest  InputSameDT=on
  Discrete-Time Integrator : DiscreteIntegrator  SampleTime=-1  ICPrevOutput=DiscIntNeverNeededParam  ICPrevScaledInput=DiscIntNeverNeededParam
  Divide : Product  Inputs=*/
  Divide1 : Product  Inputs=*/
  Product : Product
  R1 LUT : Lookup_n-D  NumberOfTableDimensions=1  BreakpointsForDimension1=msk_batt_soc_bpt  Table=msk_batt_R1  ExtrapMethod=Clip  UseLastTableValue=on  InternalRulePriority=Speed  RndMeth=Simplest  InputSameDT=on
  U_PC : Outport
  wires:
  Product/1 -> Divide1/2
  SOC/1 -> R1 LUT/1, C1 LUT/1
  Divide1/1 -> Add1/1
  C1 LUT/1 -> Product/2, Divide/2
  Divide/1 -> Add1/2
  R1 LUT/1 -> Product/1
  Discrete-Time Integrator/1 -> U_PC/1, Divide1/1  "U_PC"
  Add1/1 -> Discrete-Time Integrator/1  "U_PC_derivative"
  Current/1 -> Divide/1

== system platooning_custom_blocks/Series Parallel Hybrid Electric Truck/Series Parallel Hybrid Electric Powertrain Power Loss Model/A123 ESS Model/R2_C2 Circuit ==
  SOC : Inport
  Current : Inport  Port=2
  Add1 : Sum
  C2 LUT : Lookup_n-D  NumberOfTableDimensions=1  BreakpointsForDimension1=msk_batt_soc_bpt  Table=msk_batt_C2  ExtrapMethod=Clip  UseLastTableValue=on  InternalRulePriority=Speed  RndMeth=Simplest  InputSameDT=on
  Discrete-Time Integrator : DiscreteIntegrator  SampleTime=-1  ICPrevOutput=DiscIntNeverNeededParam  ICPrevScaledInput=DiscIntNeverNeededParam
  Divide : Product  Inputs=*/
  Divide1 : Product  Inputs=*/
  Product : Product
  R2 LUT : Lookup_n-D  NumberOfTableDimensions=1  BreakpointsForDimension1=msk_batt_soc_bpt  Table=msk_batt_R2  ExtrapMethod=Clip  UseLastTableValue=on  InternalRulePriority=Speed  RndMeth=Simplest  InputSameDT=on
  U_PA : Outport
  wires:
  Product/1 -> Divide1/2
  SOC/1 -> R2 LUT/1, C2 LUT/1
  Divide1/1 -> Add1/1
  C2 LUT/1 -> Product/2, Divide/2
  Divide/1 -> Add1/2
  R2 LUT/1 -> Product/1
  Discrete-Time Integrator/1 -> U_PA/1, Divide1/1  "U_PA"
  Add1/1 -> Discrete-Time Integrator/1  "U_PA_derivative"
  Current/1 -> Divide/1

== system platooning_custom_blocks/Series Parallel Hybrid Electric Truck/Series Parallel Hybrid Electric Powertrain Power Loss Model/Electric Drivetrain/Motor Fault Injection ==
  MOT_SPD_IN : Inport
  P_ELEC : Inport  Port=2
  Clock : Inport  Port=3
  Add : Sum  Inputs=|-+
  Add1 : Sum
  Constant : Constant  Value=t_fault
  Constant1 : Constant  Value=0
  Constant2 : Constant  Value=contMotTrqMax
  Delay : Delay  DelayLength=1
  Discrete PID Controller : simulink/Continuous/PID Controller  Controller=PI  Form=Parallel  TimeDomain=Discrete-time  SampleTime=-1  IntegratorMethod=Forward Euler  FilterMethod=Forward Euler  ControllerParametersSource=internal  P=0.002  I=0.003  D=0  UseFilter=on  N=100  TunerSelectOption=Transfer Function Based (PID Tuner App)  InitialConditionSource=internal  InitialConditionForIntegrator=0  InitialConditionForFilter=0  DifferentiatorICPrevScaledInput=0  ExternalReset=none  TrackingMode=off  Kt=1  LimitOutput=on  UpperSaturationLimit=0  LowerSaturationLimit=-inf  LinearizeAsGain=off  AntiWindupMode=clamping  Kb=1  POutMin=[]  POutMax=[]  IOutMin=[]  IOutMax=[]  DOutMin=[]  DOutMax=[]  NOutMin=[]  NOutMax=[]  SumOutMin=[]  SumOutMax=[]  SaturationOutMin=[]  SaturationOutMax=[]  PParamMin=[]  PParamMax=[]  IParamMin=[]  IParamMax=[]  DParamMin=[]  DParamMax=[]  NParamMin=[]  NParamMax=[]  KbParamMin=[]  KbParamMax=[]  KtParamMin=[]  KtParamMax=[]  KbOutMin=[]  KbOutMax=[]  KtOutMin=[]  KtOutMax=[]  IntegratorOutMin=[]  IntegratorOutMax=[]  FilterOutMin=[]  FilterOutMax=[]  SumI1OutMin=[]  SumI1OutMax=[]  SumI2OutMin=[]  SumI2OutMax=[]  SumI3OutMin=[]  SumI3OutMax=[]  SumI4OutMin=[]  SumI4OutMax=[]  SumDOutMin=[]  SumDOutMax=[]  DifferentiatorOutMin=[]  DifferentiatorOutMax=[]  FilterDiffOutCoefMin=[]  FilterDiffOutCoefMax=[]  ReciprocalOutMin=[]  ReciprocalOutMax=[]  SumDenOutMin=[]  SumDenOutMax=[]  SumNumOutMin=[]  SumNumOutMax=[]  DivideOutMin=[]  DivideOutMax=[]  IntegratorContinuousStateAttributes=''  IntegratorStateMustResolveToSignalObject=off  IntegratorRTWStateStorageClass=Auto  FilterContinuousStateAttributes=''  FilterStateMustResolveToSignalObject=off  FilterRTWStateStorageClass=Auto  ParallelPVariant=InternalParameters  IdealPVariant=Disabled  IVariant=InternalParameters  DVariant=Disabled  IntegratorVariant=Discrete  SatVariant=Enabled  AWVariant=DiscClampingParallel  PCopyVariant=Disabled  TRVariant=Disabled  FdbkBlocksVariant=Forward  IdealPFdbkVariant=Disabled  SatFdbkVariant=Disabled  DerivativeFilterVariant=Disabled  NVariant=Disabled  NCopyVariant=Disabled_SignalSpec  FilterICVariant=Disabled  IntegratorICVariant=InternalICs  ExternalResetVariant=Disabled  TRSumVariant=Passthrough  SumFdbkVariant=Disabled  SumVariant=Sum_PI
  Divide : Product  Inputs=*/
  Equal : RelationalOperator  OutDataTypeStr=boolean  RndMeth=Simplest
  Fault Assertion : Assertion  Commented=on  AssertionFailFcn=|  StopWhenAssertionFail=off
      | set_param(bdroot,'SimulationCommand','pause');
      | disp('## Paused due to Motor fault insertion')
  Gain : Gain  Gain=2
  Logic : Stateflow chart  TreatAsAtomicUnit=on
  Multiport Switch : MultiPortSwitch  DataPortOrder=Zero-based contiguous  Inputs=2  zeroidx=on
  P_ref : Constant  Value=P_derate/2
  P_ref1 : Constant  Value=inf
  Saturation Dynamic : simulink/Discontinuities/Saturation Dynamic  OutMin=[]  OutMax=[]  OutDataTypeStr=Inherit: Same as second input  OutDataType=fixdt(1, 16)  OutScaling=2^-10  DoSatur=off
  Switch : Switch  Criteria=u2 > Threshold
  Switch1 : Switch  Criteria=u2 > Threshold
  choice : Constant  Value=FaultDec
  MOT_SPD_OUT : Outport
  wires:
  Multiport Switch/1 -> MOT_SPD_OUT/1  "omega_mot_radps"
  choice/1 -> Logic/2(choice), Multiport Switch/1
  Add/1 -> Discrete PID Controller/1
  P_ELEC/1 -> Delay/1
  Delay/1 -> Add/1
  Discrete PID Controller/1 -> Add1/2  "PI_Out"
  MOT_SPD_IN/1 -> Multiport Switch/2, Add1/1
  P_ref/1 -> Gain/1, Switch/1
  Saturation Dynamic/1 -> Multiport Switch/3  "omega_mot_radps"
  Add1/1 -> Saturation Dynamic/2  "omega_mot_radps"
  Clock/1 -> Equal/1
  Constant/1 -> Equal/2
  Equal/1 -> Logic/1(input), Switch1/2, Switch/2
  Switch/1 -> Add/2
  P_ref1/1 -> Switch1/3, Switch/3
  Constant1/1 -> Saturation Dynamic/3
  Gain/1 -> Divide/1
  Constant2/1 -> Divide/2
  Divide/1 -> Switch1/1  "max_omega_derate"
  Switch1/1 -> Saturation Dynamic/1
  Logic/1(trigger) -> Fault Assertion/1  "faultTrigger"

== matlab function platooning_custom_blocks/Conventional Truck Driver and Vehicle Acceleration Dynamics Model/Gear Shift Logic ==
  data: upshift_req input; gear_cmd output; dnshift_req input; init_gear input; gear_ratio output; gear_rat_vec input
function [gear_cmd, gear_ratio] = fcn(upshift_req, dnshift_req, init_gear, gear_rat_vec)
    % Standard LUT based gear switch logic
    %% Pre-processing
    persistent prev_gear
    if isempty(prev_gear)
        prev_gear = init_gear;
    end
    temp_gear = prev_gear;                  % If no change in gear.
    len = length(gear_rat_vec);             % One-based idexing for gears
    
    %% Gear Shift Logic
    if temp_gear > 1 && temp_gear < len
        if upshift_req == 1
            temp_gear = temp_gear + 1;
        elseif dnshift_req == 1
            temp_gear = temp_gear - 1;
        end
    elseif temp_gear == 1
        if upshift_req == 1
            temp_gear = temp_gear + 1;
        end
    elseif temp_gear == len
        if dnshift_req == 1
            temp_gear = temp_gear - 1;
        end
    end
    %% Post-processing
    gear_cmd = temp_gear;
    gear_ratio = gear_rat_vec(temp_gear);
    prev_gear = temp_gear;
 
end

== matlab function platooning_custom_blocks/2 DOF Longitudinal Dynamics Model - Force Input/2 DOF Longitudinal Dynamics Model - Force Input ==
  data: F_prop input; veh_spd_out output; alpha_grd input; x_sep input; v_init input; msk_tstep input; msk_mass input; msk_rho_air input; msk_Af input; msk_Cd input; msk_r_tire input; msk_roadType input; veh_acc_ms2 output; F_prop output; F_ar output; F_cr output; F_rr output; P_prop output; P_ar output; P_cr output; P_rr output
function [veh_spd_out, veh_acc_ms2, F_prop, F_ar, F_cr, F_rr, P_prop, P_ar, P_cr, P_rr] = ...
    lngdyn_2dof_finp(F_prop, alpha_grd, x_sep, v_init, msk_tstep, msk_mass, msk_rho_air,...
    msk_Af, msk_Cd, msk_r_tire, msk_roadType)
% LNGDYN_2DOF 2 DOF Longitudinal Dynamics Model
%   This model focues on two degrees of freedom i.e. longitudinal
%   translation and pitch movement. The force equation is used to compute
%   the power demand by the vehicle for propulsion.
%   INPUT ARGUMENTS:
%   --> F_prop:         Propulsive force [N]
%   --> alpha_grd:      Road grade percentage [%]  
%   --> x_sep:          Inter-vehicle separation distance for Cd variation [m]
%   --> v_init:         Initial speed [m/s]
%   --> msk_tstep:      Masked Value - time step [sec]
%   --> msk_mass:       Masked Value - vehicle mass [kg]
%   --> msk_rho_air:    Masked Value - air density [kg/m3]
%   --> msk_Af:         Masked Value - frontal area [m2]
%   --> msk_Cd:         Masked Value - Coefficient of drag [-]
%   --> msk_r_tire:     Masked Value - tire radius [m]
%   --> msk_roadType:   Masked Value - type of road for road resistance
%   coefficients [enum]
%   OUTPUT ARGUMENTS:
%   --> veh_spd_out:        Vehicle speed [m/s]
%   --> veh_acc_ms2:    Vehicle acceleration [m/s^2]
%   --> F_ar:           Aerodynamic force [N]
%   --> F_cr:           Climbing force [N]
%   --> P_prop:         Propulsuve power [W]
%   --> P_ar:           Aerodynamic power [W]
%   --> P_cr:           Climbing power [W]


%% Pre-processing
persistent v_old
if isempty(v_old)
    v_old = v_init;
end
g = 9.81;
alp_frac = alpha_grd/100;
% -- Road Type based Coefficient Variation --
% Assumed Radial Tyres - Only for Trucks
switch msk_roadType
    case 0
        C_h = 1.0;
    case 1
        C_h = 1.2;
    case 2
        C_h = 1.5;
    otherwise
        C_h = 1.0;
end
%% Road Load Calculation - Solve for v[k]: a.v^2 + b.v + c = 0
a = 0.5 * msk_rho_air * msk_Af * msk_Cd;
b = (msk_mass/msk_tstep) + (0.000041 * 2.23694 * C_h * msk_mass * g * cos(alp_frac));
c = -1 * (F_prop - (msk_mass * g * sin(alp_frac)) - ...
    (0.0041 * msk_mass * g * cos(alp_frac)) + ((msk_mass/msk_tstep) * v_old));
v_roots = zeros([2 1]);
v_roots = real(roots([a b c]));

if v_roots(1) >= 0 && v_roots(2) < 0
    veh_spd_out = v_roots(1);
elseif v_roots(1) < 0 && v_roots(2) >= 0
    veh_spd_out = v_roots(2);
elseif (v_roots(1) == v_roots(2)) && (v_roots(1) >= 0)
    veh_spd_out = v_roots(1);
else
    veh_spd_out = 0;
end

% -- Acceleration Calculation --
veh_acc_ms2 = (veh_spd_out - v_old)/msk_tstep;
%% Resistance Force Calculations
F_ar = 0.5 * msk_rho_air * msk_Af * msk_Cd * (veh_spd_out^2);
F_cr = msk_mass * g * sin(alp_frac);
F_rr = ((0.0041 + (0.000041 * veh_spd_out * 2.23694)) * C_h) * msk_mass * g * cos(alp_frac);
F_prop = (msk_mass * veh_acc_ms2) + F_ar + F_cr + F_rr;

%% Resistance Power Calculations
P_ar = F_ar * veh_spd_out;
P_cr = F_cr * veh_spd_out;
P_prop = F_prop * veh_spd_out;
P_rr = F_rr * veh_spd_out;


%% Post-processing
v_old = veh_spd_out;
end

== matlab function platooning_custom_blocks/2 DOF Longitudinal Dynamics Model - Speed Input/2DOF Longitudinal Dynamics Model - Speed Input ==
  data: veh_acc_ms2 output; v_spd input; F_prop output; alpha_grd input; x_sep input; msk_tstep input; msk_mass input; msk_rho_air input; msk_Af input; msk_Cd input; msk_r_tire input; msk_roadType input; F_ar output; F_cr output; P_prop output; P_ar output; P_cr output
function [veh_acc_ms2, F_prop, F_ar, F_cr, P_prop, P_ar, P_cr] = ...
    lngdyn_2dof(v_spd, alpha_grd, x_sep, msk_tstep, msk_mass, msk_rho_air,...
    msk_Af, msk_Cd, msk_r_tire, msk_roadType)
% LNGDYN_2DOF 2 DOF Longitudinal Dynamics Model
%   This model focues on two degrees of freedom i.e. longitudinal
%   translation and pitch movement. The force equation is used to compute
%   the power demand by the vehicle for propulsion.
%   OUTPUT ARGUMENTS:
%   --> F_prop: Propulsive force [N]
%   --> F_ar:   Aerodynamic force [N]
%   --> F_cr:   Climbing force [N]
%   --> P_prop: Propulsuve power [W]
%   --> P_ar:   Aerodynamic power [W]
%   --> P_cr:   Climbing power [W]
%   INPUT ARGUMENTS:
%   --> v_spd:      Vehicle speed input [m/s]
%   --> alpha_grd:  Road grade percentage [%]  
%   --> x_sep:      Inter-vehicle separation distance for Cd variation [m]
%   --> msk_tstep:  Masked Value - time step [sec]
%   --> msk_mass:   Masked Value - vehicle mass [kg]
%   --> msk_rho_air:Masked Value - air density [kg/m3]
%   --> msk_Af:     Masked Value - frontal area [m2]
%   --> msk_Cd:     Masked Value - Coefficient of drag [-]
%   --> msk_r_tire: Masked Value - tire radius [m]
%   --> msk_roadType:   Masked Value - type of road for road resistance
%   coefficients [enum]

%% Pre-processing
persistent v_spd_old
if isempty(v_spd_old)
    v_spd_old = v_spd;
end
g = 9.81;
alp_frac = alpha_grd/100;
% -- Road Type based Coefficient Variation --
% Assumed Radial Tyres - Only for Trucks
switch msk_roadType
    case 0
        C_h = 1.0;
    case 1
        C_h = 1.2;
    case 2
        C_h = 1.5;
    otherwise
        C_h = 1.0;
end
% -- Acceleration Calculation --
veh_acc_ms2 = (v_spd - v_spd_old)/msk_tstep;
%% Resistance Force Calculations
F_ar = 0.5 * msk_rho_air * msk_Af * msk_Cd * (v_spd^2);
F_cr = msk_mass * g * sin(alp_frac);
F_rr = ((0.0041 + (0.000041 * v_spd * 2.23694)) * C_h) * msk_mass * g * cos(alp_frac);
F_prop = (msk_mass * veh_acc_ms2) + F_ar + F_cr + F_rr;

%% Resistance Power Calculations
P_ar = F_ar * v_spd;
P_cr = F_cr * v_spd;
P_prop = F_prop * v_spd;

%% Post - Processing
v_spd_old = v_spd;

end

== matlab function platooning_custom_blocks/Series Parallel Hybrid Electric Truck Driver and Vehicle Acceleration Dynamics Model - Force Output/Gear Shift Logic ==
  data: upshift_req input; gear_cmd output; dnshift_req input; init_gear input; gear_ratio output; gear_rat_vec input
function [gear_cmd, gear_ratio] = fcn(upshift_req, dnshift_req, init_gear, gear_rat_vec)
    % Standard LUT based gear switch logic
    %% Pre-processing
    persistent prev_gear
    if isempty(prev_gear)
        prev_gear = init_gear;
    end
    temp_gear = prev_gear;                  % If no change in gear.
    len = length(gear_rat_vec);             % One-based idexing for gears
    
    %% Gear Shift Logic
    if temp_gear > 1 && temp_gear < len
        if upshift_req == 1
            temp_gear = temp_gear + 1;
        elseif dnshift_req == 1
            temp_gear = temp_gear - 1;
        end
    elseif temp_gear == 1
        if upshift_req == 1
            temp_gear = temp_gear + 1;
        end
    elseif temp_gear == len
        if dnshift_req == 1
            temp_gear = temp_gear - 1;
        end
    end
    %% Post-processing
    gear_cmd = temp_gear;
    gear_ratio = gear_rat_vec(temp_gear);
    prev_gear = temp_gear;
 
end

== matlab function platooning_custom_blocks/Conventional Truck/Conventional Powertrain Power Loss Model/AWGN Function ==
  data: inp input; out output; snr input
function out = addnoise(inp,snr)

out = awgn(inp,snr,'measured');
